simulink model "secondweekfourth"  (R2020a)
settings: Solver=VariableStepAuto  StartTime=0.0  StopTime=10.0  RelTol=1e-3
model workspace (MAT data in the model file):
  J = Simulink.Parameter
  J.Value = 3.2284e-06
  J.DataType = 'auto'
  J.Dimensions = [1 1]
  K = Simulink.Parameter
  K.Value = 0.0274
  K.DataType = 'auto'
  K.Dimensions = [1 1]
  Kd = Simulink.Parameter
  Kd.Value = 50
  Kd.DataType = 'auto'
  Kd.Dimensions = [1 1]
  Ki = Simulink.Parameter
  Ki.Value = 300
  Ki.DataType = 'auto'
  Ki.Dimensions = [1 1]
  Kp = Simulink.Parameter
  Kp.Value = 350
  Kp.DataType = 'auto'
  Kp.Dimensions = [1 1]
  L = Simulink.Parameter
  L.Value = 2.75
  L.DataType = 'auto'
  L.Dimensions = [1 1]
  R = Simulink.Parameter
  R.Value = 4
  R.DataType = 'auto'
  R.Dimensions = [1 1]
  b = Simulink.Parameter
  b.Value = 3.5077e-06
  b.DataType = 'auto'
  b.Dimensions = [1 1]
settings Model: DataDictionary=datadict.sldd  Creator=Admin  LastModifiedBy=Admin

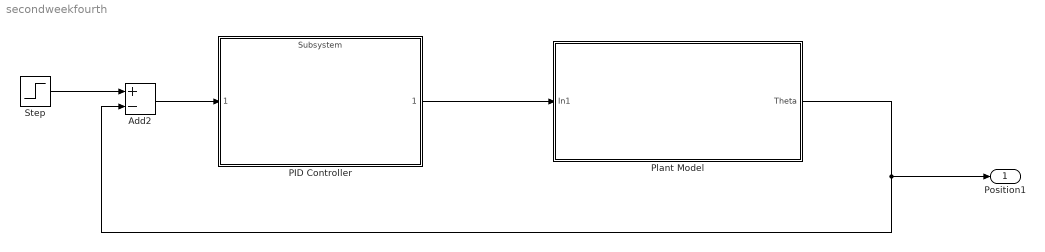
== system secondweekfourth ==
  Add2 : Sum  Inputs=+-
  PID Controller : ModelReference  ModelNameDialog=Subsystem  ModelReferenceVersion=1.14
  Plant Model : Subsystem
  Step : Step  Time=0.1  SampleTime=0
  Position1 : Outport
  wires:
  Step/1 -> Add2/1
  Add2/1 -> PID Controller/1
  Plant Model/1(Theta) -> Add2/2, Position1/1
  PID Controller/1 -> Plant Model/1(In1)

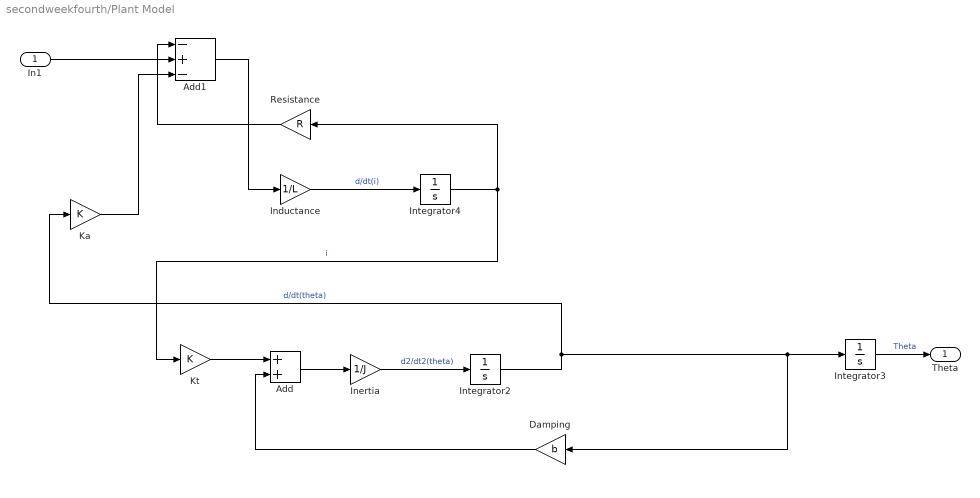
== system secondweekfourth/Plant Model ==
  In1 : Inport
  Add : Sum
  Add1 : Sum  Inputs=-+-
  Damping : Gain  Gain=b
  Inductance : Gain  Gain=1/L
  Inertia : Gain  Gain=1/J
  Integrator2 : Integrator
  Integrator3 : Integrator
  Integrator4 : Integrator
  Ka : Gain  Gain=K
  Kt : Gain  Gain=K
  Resistance : Gain  Gain=R
  Theta : Outport
  wires:
  Integrator3/1 -> Theta/1  "Theta"
  Integrator4/1 -> Kt/1, Resistance/1  "i"
  Kt/1 -> Add/1
  Resistance/1 -> Add1/1
  In1/1 -> Add1/2
  Ka/1 -> Add1/3
  Inductance/1 -> Integrator4/1  "d/dt(i)"
  Integrator2/1 -> Integrator3/1, Damping/1, Ka/1  "d/dt(theta)"
  Add/1 -> Inertia/1
  Add1/1 -> Inductance/1
  Damping/1 -> Add/2
  Inertia/1 -> Integrator2/1  "d2/dt2(theta)"
